simulink model "wind_simulink_constr_1"  (R2023b)
settings: Solver=VariableStepAuto  StartTime=0.0  StopTime=30  RelTol=1e-3
values from neighbouring files (symbols this model uses):
  pole_lpf = 0.005    [WindTurbine_MPC.m]
  Ts = 0.005    [WindTurbine_MPC.m]
libraries: simulink x2
settings Model: Creator=marco  LastModifiedBy=marco
settings OptimizationCC: ReuseModelBlockBuffer=off

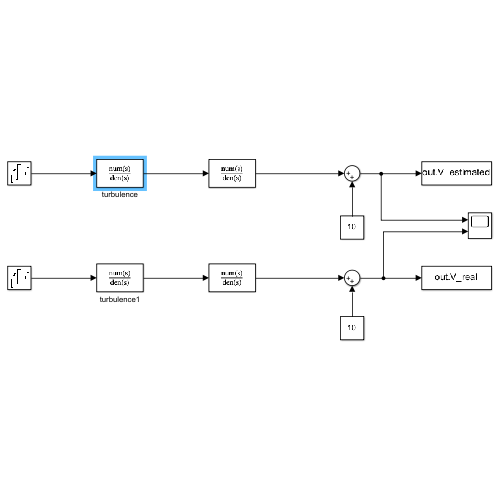
[thumbnail: Simulink's stored preview of the top-level diagram]
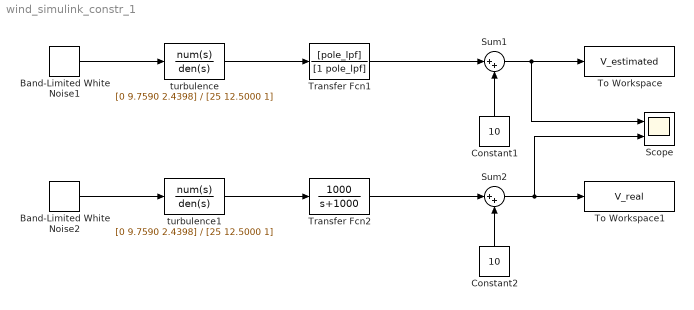
== system wind_simulink_constr_1 ==
  Band-Limited White Noise1 : simulink/Sources/Band-Limited White Noise  Cov=[5]  Ts=Ts  seed=[23341]
  Band-Limited White Noise2 : simulink/Sources/Band-Limited White Noise  Cov=[5]  Ts=Ts  seed=[23341]
  Constant1 : Constant  Value=10  VectorParams1D=off
  Constant2 : Constant  Value=10  VectorParams1D=off
  Scope : Scope  NumInputPorts=2
  Sum1 : Sum  Inputs=|++
  Sum2 : Sum  Inputs=|++
  To Workspace : ToWorkspace  VariableName=V_estimated  SampleTime=Ts
      settings: Save2DSignal=2-D array (concatenate along first dimension)
  To Workspace1 : ToWorkspace  VariableName=V_real  SampleTime=Ts
      settings: Save2DSignal=2-D array (concatenate along first dimension)
  Transfer Fcn1 : TransferFcn  Numerator=[pole_lpf]  Denominator=[1 pole_lpf]
  Transfer Fcn2 : TransferFcn  Numerator=[1000]  Denominator=[1 1000]
  turbulence : TransferFcn  Numerator=[0 9.7590 2.4398]  Denominator=[25 12.5000 1]
  turbulence1 : TransferFcn  Numerator=[0 9.7590 2.4398]  Denominator=[25 12.5000 1]
  wires:
  Band-Limited White Noise1/1 -> turbulence/1
  turbulence/1 -> Transfer Fcn1/1
  Constant1/1 -> Sum1/2
  Sum1/1 -> Scope/1, To Workspace/1
  Transfer Fcn1/1 -> Sum1/1
  Band-Limited White Noise2/1 -> turbulence1/1
  turbulence1/1 -> Transfer Fcn2/1
  Constant2/1 -> Sum2/2
  Transfer Fcn2/1 -> Sum2/1
  Sum2/1 -> To Workspace1/1, Scope/2
